simulink model "s2dot2_57yihuo"  (R2023b)
settings: Solver=VariableStepAuto  StartTime=0.0  StopTime=10.0  RelTol=1e-3
settings Model: Creator=lxj  LastModifiedBy=lxj

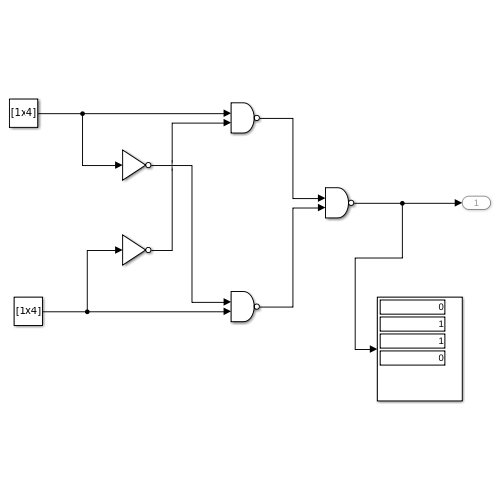
[thumbnail: Simulink's stored preview of the top-level diagram]
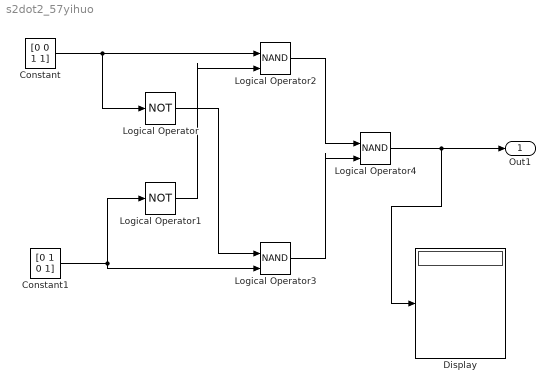
== system s2dot2_57yihuo ==
  Constant : Constant  Value=[0 0 1 1]
  Constant1 : Constant  Value=[0 1 0 1]
  Display : Display
  Logical Operator : Logic  Operator=NOT  IconShape=distinctive  AllPortsSameDT=off  OutDataTypeStr=boolean
  Logical Operator1 : Logic  Operator=NOT  IconShape=distinctive  AllPortsSameDT=off  OutDataTypeStr=boolean
  Logical Operator2 : Logic  Operator=NAND  IconShape=distinctive  AllPortsSameDT=off  OutDataTypeStr=boolean
  Logical Operator3 : Logic  Operator=NAND  IconShape=distinctive  AllPortsSameDT=off  OutDataTypeStr=boolean
  Logical Operator4 : Logic  Operator=NAND  IconShape=distinctive  AllPortsSameDT=off  OutDataTypeStr=boolean
  Out1 : Outport
      settings: EnsureOutportIsVirtual=on
  wires:
  Constant/1 -> Logical Operator/1, Logical Operator2/1
  Constant1/1 -> Logical Operator1/1, Logical Operator3/2
  Logical Operator/1 -> Logical Operator3/1
  Logical Operator1/1 -> Logical Operator2/2
  Logical Operator2/1 -> Logical Operator4/1
  Logical Operator3/1 -> Logical Operator4/2
  Logical Operator4/1 -> Display/1, Out1/1
